simulink model "mdaqdemo_tsend"  (R2013a)
settings: Solver=FixedStepDiscrete  SolverMode=SingleTasking  StartTime=0.0  StopTime=inf  FixedStep=0.1  RelTol=1e-3
libraries: microdaq_lib x1
settings Model: Creator=peselnikmg  LastModifiedBy=skibool
settings DataIOCC: SignalLoggingSaveFormat=ModelDataLogs
settings OptimizationCC: OptimizeModelRefInitCode=on  LifeSpan=1
settings DebuggingCC: MultiTaskDSMMsg=warning  MultiTaskCondExecSysMsg=none  StateNameClashWarn=none  StrictBusMsg=None
settings HardwareCC: ProdBitPerLong=40  ProdLargestAtomicInteger=Integer  ProdIntDivRoundTo=Zero  ProdEndianess=LittleEndian  ProdHWDeviceType=Texas Instruments->C6000
settings RTWCC: SystemTargetFile=microdaq.tlc  TemplateMakefile=microdaq.tmf  PostCodeGenCommand=microdaq_postcodegen(buildInfo)  Description=MicroDAQ Real-Time Measurement System  GenerateReport=on  ProcessScript=microdaq_make_rtw_hook  IncludeHyperlinkInReport=on  LaunchReport=on  IncludeERTFirstTime=on  GenerateTraceInfo=on  GenerateTraceReport=on  GenerateTraceReportSl=on  GenerateTraceReportSf=on  GenerateTraceReportEml=on
settings CodeAppCC: IgnoreCustomStorageClasses=off
settings STFCustomTargetCC: CodeReplacementLibrary=TI C674x  CombineOutputUpdateFcns=on  ERTCustomFileBanners=on  SupportContinuousTime=off  SupportNonInlinedSFcns=off  MATLABClassNameForMDSCustomization=Simulink.SoftwareTarget.ERTCustomization  SystemTargetFile=microdaq.tlc
settings ERTTargetCC: CodeReplacementLibrary=TI C674x  GenerateSampleERTMain=off  ParMdlRefBuildCompliant=off  CompOptLevelCompliant=off  ConcurrentExecutionCompliant=off  ERTFirstTimeCompliant=off  ModelStepFunctionPrototypeControlCompliant=off  CPPClassGenCompliant=off  ExtModeStaticAlloc=on  ExtModeStaticAllocSize=10485760  ExtModeMexArgs=getpref('microdaq','TargetIP') 1 4344  ERTCustomFileTemplate=microdaq_main.tlc

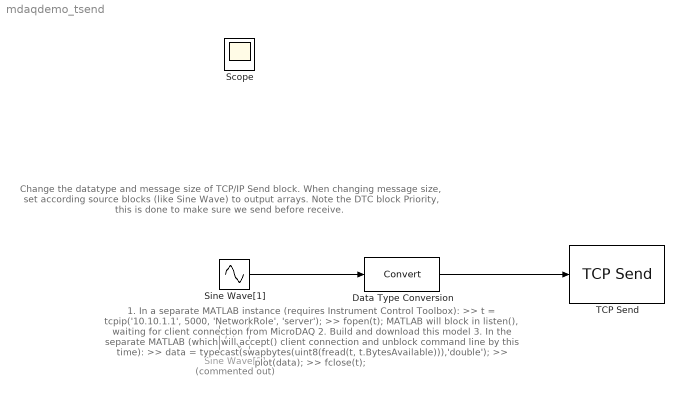
== system mdaqdemo_tsend ==
  note: 1. In a separate MATLAB instance (requires Instrument Control Toolbox):
      | >> t = tcpip('10.10.1.1', 5000, 'NetworkRole', 'server');
      | >> fopen(t);
      | MATLAB will block in listen(), waiting for client connection from MicroDAQ
      |
      | 2. Build and download this model
      | 3. In the separate MATLAB (which will accept() client
      | connection and unblock command line by this time):
      | >> data = typecast(swapbytes(uint8(fread(t, t.BytesAvailable))),'double');
      | >> plot(data);
      | >> fclose(t);
  note: Change the datatype and message size of TCP/IP Send block.
      | When changing message size, set according source blocks (like Sine Wave) to output arrays.
      | Note the DTC block Priority, this is done to make sure we send before receive.
  Data Type Conversion : DataTypeConversion  Priority=1
      settings: AttributesFormatString=Priority: %<Priority>
  Sine Wave[1] : Sin
  Sine Wave[2] : Sin  Commented=on  Amplitude=[1 2]
  TCP Send : microdaq_lib/Network/TCP Send  IPAddrStr='10.10.1.10'  Port=5000  Blocking=off  Timeout=250  Datatype=double  SizePack=1  SampleTime=-1
  Scope : Scope
  wires:
  Data Type Conversion/1 -> TCP Send/1
  Sine Wave[1]/1 -> Data Type Conversion/1
